simulink model "dspwdnoisfp"  (Simulink 6.0)
settings: Solver=FixedStepDiscrete  SolverMode=SingleTasking  StartTime=0.0  StopTime=1024  RelTol=1e-3
PreLoadFcn:
  | load dspwlets;
values from neighbouring files (symbols this model uses):
  ts = get_param(blk,'CompiledSampleTime')    [sdspwwvdisp.m]
undefined symbols (not defined in the file or in its folder): hid, hir, lod, lor
libraries: dspmlti4 x6, dspsigops x3, dspsrcs4 x1
settings Model: Creator=don  LastModifiedBy=schim  ExtModeTrigMode=oneshot  ExtModeArmWhenConnect=off
settings DataIOCC: LimitDataPoints=off  SaveOutput=off  SaveTime=off  SignalLoggingName=sigsOut
settings OptimizationCC: BlockReduction=off  BooleanDataType=off  MultiInstanced=off
settings FormatCC: IgnoreBidirectionalLines=off
settings DebuggingCC: IntegerOverflowMsg=none  ParameterPrecisionLossMsg=none
settings HardwareCC: TargetUnknown=on
settings CodeAppCC: SimulinkBlockComments=off
settings GRTTargetCC: TargetFcnLib=iso_c_tmw.mat

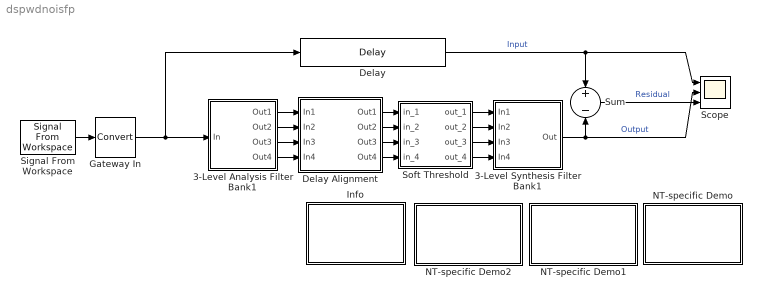
== system dspwdnoisfp ==
  3-Level Analysis Filter Bank1 : Subsystem  mask{low=lod, high=hid}
      mask prompts: low "Lowpass FIR filter coefficients:"; high "Highpass FIR filter coefficients:"
  3-Level Synthesis Filter Bank1 : Subsystem  mask{low=lor, high=hir}
      mask prompts: low "Lowpass FIR filter coefficients:"; high "Highpass FIR filter coefficients:"
  Delay : dspsigops/Delay  dly_unit=Samples  delay=7*(length(lod)-1)  ic_detail=on  dif_ic_for_ch=off  dif_ic_for_dly=off  ic=0  reset_popup=None
  Delay Alignment : Subsystem
  Gateway In : DataTypeConversion  OutDataTypeMode=Specify via dialog  OutScaling=2^-10  RndMeth=Nearest  SaturateOnIntegerOverflow=on
  Info : Subsystem
      mask Type: Frame-Based Simulation Info
      mask Display: disp('Info')
  NT-specific Demo : Subsystem
      settings: OpenFcn=dspwdnoisf_win32
      mask Type: NT-only Demo
      mask Display: disp('PC/Windows\nDemo')
  NT-specific Demo1 : Subsystem
      settings: OpenFcn=dspwdnoisf
      mask Type: Frame-Based Demo
      mask Display: disp('Frame-Based\nDemo')
  NT-specific Demo2 : Subsystem
      settings: OpenFcn=dspwdnois
      mask Type: Sample-Based Demo
      mask Display: disp('Sample-Based\nDemo')
  Scope : Scope  NumInputPorts=3
      settings: TimeRange=1025  YMin=-10~-10~-5  YMax=10~10~5
  Signal From Workspace : dspsrcs4/Signal From Workspace  X=noisdopp  Ts=ts  nsamps=1  OutputAfterFinalValue=Setting to zero
  Soft Threshold : Subsystem  mask(Soft Threshold){st=[3 2 1 0]}
      mask prompts: st "Vector of thresholds for each level:"
      mask help: Apply a soft threshold (deadzone transfer function) to each signal in the decomposition. First threshold applies to top-most filter bank output.
      mask init:
      | x=([-1 1 NaN 0 0 NaN -1 -.5 .5 1]+1)/2*.7+.15;
      | y=([0 0 NaN -1 1 NaN -1 0 0 1]+1)/2*.7+.05;
      mask Help: Vector of thresholds for each decomposition level.
      mask Display:
      | text(.1,.9,'Dead Zone')
      | plot(x,y)
  Sum : Sum  Inputs=+-  SaturateOnIntegerOverflow=on  InputSameDT=on
  wires:
  Signal From Workspace/1 -> Gateway In/1
  Soft Threshold/1(out_1) -> 3-Level Synthesis Filter Bank1/1(In1)
  Soft Threshold/2(out_2) -> 3-Level Synthesis Filter Bank1/2(In2)
  Soft Threshold/3(out_3) -> 3-Level Synthesis Filter Bank1/3(In3)
  Soft Threshold/4(out_4) -> 3-Level Synthesis Filter Bank1/4(In4)
  3-Level Synthesis Filter Bank1/1(Out) -> Sum/2, Scope/2  "Output"
  Sum/1 -> Scope/3  "Residual"
  3-Level Analysis Filter Bank1/1(Out1) -> Delay Alignment/1(In1)
  3-Level Analysis Filter Bank1/2(Out2) -> Delay Alignment/2(In2)
  3-Level Analysis Filter Bank1/3(Out3) -> Delay Alignment/3(In3)
  3-Level Analysis Filter Bank1/4(Out4) -> Delay Alignment/4(In4)
  Delay Alignment/1(Out1) -> Soft Threshold/1(in_1)
  Delay Alignment/2(Out2) -> Soft Threshold/2(in_2)
  Delay Alignment/3(Out3) -> Soft Threshold/3(in_3)
  Delay Alignment/4(Out4) -> Soft Threshold/4(in_4)
  Delay/1 -> Scope/1, Sum/1  "Input"
  Gateway In/1 -> Delay/1, 3-Level Analysis Filter Bank1/1(In)

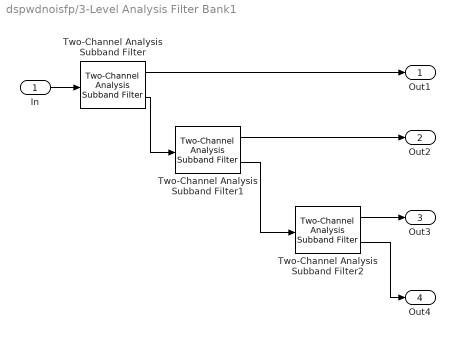
== system dspwdnoisfp/3-Level Analysis Filter Bank1 ==
  In : Inport
  Two-Channel Analysis Subband Filter : dspmlti4/Two-Channel Analysis Subband Filter  DialogController=dspDDGCreate  DialogControllerArgs=DataTag0  lpf=low  hpf=high  framing=Maintain input frame size  accumMode=Binary point scaling  accumWordLength=32  accumFracLength=25  roundingMode=Nearest  overflowMode=on
      settings: allowOverrides=off
  Two-Channel Analysis Subband Filter1 : dspmlti4/Two-Channel Analysis Subband Filter  DialogController=dspDDGCreate  DialogControllerArgs=DataTag1  lpf=low  hpf=high  framing=Maintain input frame size  accumMode=Binary point scaling  accumWordLength=32  accumFracLength=25  roundingMode=Nearest  overflowMode=on
      settings: allowOverrides=off
  Two-Channel Analysis Subband Filter2 : dspmlti4/Two-Channel Analysis Subband Filter  DialogController=dspDDGCreate  DialogControllerArgs=DataTag2  lpf=low  hpf=high  framing=Maintain input frame size  accumMode=Binary point scaling  accumWordLength=32  accumFracLength=25  roundingMode=Nearest  overflowMode=on
      settings: allowOverrides=off
  Out1 : Outport
  Out2 : Outport  Port=2
  Out3 : Outport  Port=3
  Out4 : Outport  Port=4
  wires:
  Two-Channel Analysis Subband Filter1/2 -> Two-Channel Analysis Subband Filter2/1
  Two-Channel Analysis Subband Filter2/2 -> Out4/1
  Two-Channel Analysis Subband Filter2/1 -> Out3/1
  Two-Channel Analysis Subband Filter1/1 -> Out2/1
  Two-Channel Analysis Subband Filter/2 -> Two-Channel Analysis Subband Filter1/1
  Two-Channel Analysis Subband Filter/1 -> Out1/1
  In/1 -> Two-Channel Analysis Subband Filter/1

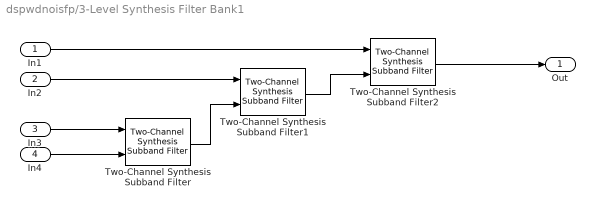
== system dspwdnoisfp/3-Level Synthesis Filter Bank1 ==
  In1 : Inport
  In2 : Inport  Port=2
  In3 : Inport  Port=3
  In4 : Inport  Port=4
  Two-Channel Synthesis Subband Filter : dspmlti4/Two-Channel Synthesis Subband Filter  DialogController=dspDDGCreate  DialogControllerArgs=DataTag3  lpf=low  hpf=high  framing=Maintain input frame size  accumMode=Binary point scaling  accumWordLength=32  accumFracLength=25  roundingMode=Nearest  overflowMode=on
      settings: allowOverrides=off
  Two-Channel Synthesis Subband Filter1 : dspmlti4/Two-Channel Synthesis Subband Filter  DialogController=dspDDGCreate  DialogControllerArgs=DataTag4  lpf=low  hpf=high  framing=Maintain input frame size  accumMode=Binary point scaling  accumWordLength=32  accumFracLength=25  roundingMode=Nearest  overflowMode=on
      settings: allowOverrides=off
  Two-Channel Synthesis Subband Filter2 : dspmlti4/Two-Channel Synthesis Subband Filter  DialogController=dspDDGCreate  DialogControllerArgs=DataTag5  lpf=low  hpf=high  framing=Maintain input frame size  accumMode=Binary point scaling  accumWordLength=32  accumFracLength=25  roundingMode=Nearest  overflowMode=on
      settings: allowOverrides=off
  Out : Outport
  wires:
  Two-Channel Synthesis Subband Filter2/1 -> Out/1
  Two-Channel Synthesis Subband Filter1/1 -> Two-Channel Synthesis Subband Filter2/2
  In1/1 -> Two-Channel Synthesis Subband Filter2/1
  Two-Channel Synthesis Subband Filter/1 -> Two-Channel Synthesis Subband Filter1/2
  In2/1 -> Two-Channel Synthesis Subband Filter1/1
  In4/1 -> Two-Channel Synthesis Subband Filter/2
  In3/1 -> Two-Channel Synthesis Subband Filter/1

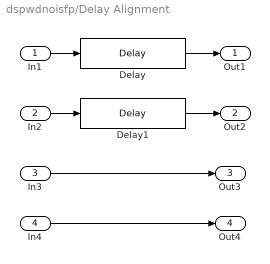
== system dspwdnoisfp/Delay Alignment ==
  In1 : Inport
  In2 : Inport  Port=2
  In3 : Inport  Port=3
  In4 : Inport  Port=4
  Delay : dspsigops/Delay  dly_unit=Samples  delay=3*(length(lod)-1)  ic_detail=on  dif_ic_for_ch=off  dif_ic_for_dly=off  ic=0  reset_popup=None
  Delay1 : dspsigops/Delay  dly_unit=Samples  delay=length(lod) - 1  ic_detail=on  dif_ic_for_ch=off  dif_ic_for_dly=off  ic=0  reset_popup=None
  Out1 : Outport
  Out2 : Outport  Port=2
  Out3 : Outport  Port=3
  Out4 : Outport  Port=4
  wires:
  In3/1 -> Out3/1
  In4/1 -> Out4/1
  In2/1 -> Delay1/1
  Delay1/1 -> Out2/1
  In1/1 -> Delay/1
  Delay/1 -> Out1/1

== system dspwdnoisfp/Info ==
  note: Demonstration of wavelet de-noising
      |
      |
      | Set the threshold levels in the "Soft Threshold" block
      | to alter the de-noising characteristics of the system:
      |
      | Threshold=[0 0 0 0]  -> No de-noising
      | (perfect reconstruction)
      |
      | Threshold=[3 2 1 0] -> Moderate de-noising
      | (removes small-scale content from signal)
      |
      |  Fixed-point version of the wavelet
      | de-noising model illustrates polyphase
      | implementations of high-pass and low-pass
      | FIR decimation filters, as shown in
      | the subsystems 3-Level Analysis Filter Bank
      | and 3-Level Synthesis Filter Bank

== system dspwdnoisfp/NT-specific Demo ==

== system dspwdnoisfp/NT-specific Demo1 ==

== system dspwdnoisfp/NT-specific Demo2 ==

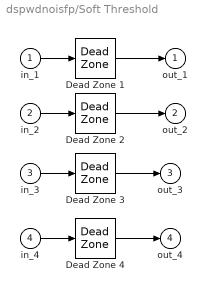
== system dspwdnoisfp/Soft Threshold ==
  in_1 : Inport
  in_2 : Inport  Port=2
  in_3 : Inport  Port=3
  in_4 : Inport  Port=4
  Dead Zone 1 : DeadZone  LowerValue=-st(1)  UpperValue=st(1)  LinearizeAsGain=off  ZeroCross=off  SaturateOnIntegerOverflow=on
  Dead Zone 2 : DeadZone  LowerValue=-st(2)  UpperValue=st(2)  LinearizeAsGain=off  ZeroCross=off  SaturateOnIntegerOverflow=on
  Dead Zone 3 : DeadZone  LowerValue=-st(3)  UpperValue=st(3)  LinearizeAsGain=off  ZeroCross=off  SaturateOnIntegerOverflow=on
  Dead Zone 4 : DeadZone  LowerValue=-st(4)  UpperValue=st(4)  LinearizeAsGain=off  ZeroCross=off  SaturateOnIntegerOverflow=on
  out_1 : Outport  InitialOutput=0
  out_2 : Outport  Port=2  InitialOutput=0
  out_3 : Outport  Port=3  InitialOutput=0
  out_4 : Outport  Port=4  InitialOutput=0
  wires:
  in_1/1 -> Dead Zone 1/1
  Dead Zone 1/1 -> out_1/1
  in_2/1 -> Dead Zone 2/1
  Dead Zone 2/1 -> out_2/1
  in_3/1 -> Dead Zone 3/1
  Dead Zone 3/1 -> out_3/1
  in_4/1 -> Dead Zone 4/1
  Dead Zone 4/1 -> out_4/1
